simulink model "example_quaternion_KF_EKF"  (R2016a)
settings: Solver=VariableStepAuto  StartTime=0.0  StopTime=25  RelTol=1e-3
values from neighbouring files (symbols this model uses):
  filterMat = filterMat(filterPlot,:)    [init.m]
  KF_C = KF_C([3,4,5,7,8,9,10,11,12,13],:)    [init.m]
  KF_mean = zeros(13,1)    [init.m]
  KF_variance = diag([0.00025, 0.049,0.049,0.05, 0.05, 0.05, 0.05, 0.005, 0.005,0.005])    [init.m]
  measureMat = measureMat(measurePlot,:)    [init.m]
undefined symbols (not defined in the file or in its folder): g, inner_h, k, m
settings Model: Creator=Daniel  LastModifiedBy=mgreiff
settings DataIOCC: LimitDataPoints=on
settings DebuggingCC: AllowSymbolicDim=off
settings ModelReferenceCC: PropagateSignalLabelsOutOfModel=off
settings GRTTargetCC: GeneratePreprocessorConditionals=Use local settings

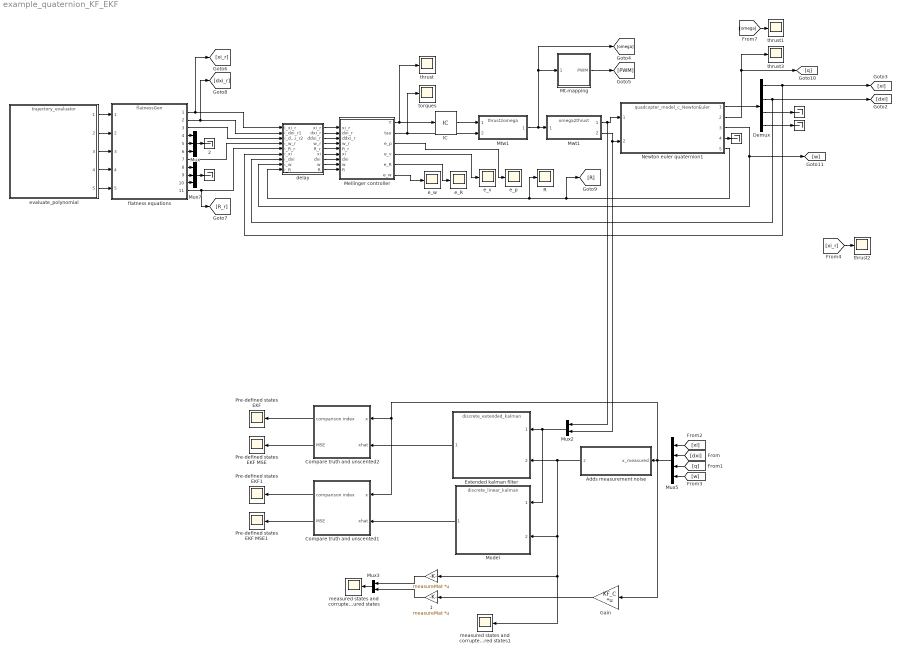
== system example_quaternion_KF_EKF ==
  " " : Gain  Gain=measureMat  Multiplication=Matrix(K*u)
  "  " : Terminator
  "     " : Terminator
  "      " : Terminator
  "       " : Terminator
  " 1" : Gain  Gain=measureMat  Multiplication=Matrix(K*u)
  " 2" : Terminator
  Adds measurement noise : Subsystem
  Compare truth and unscented1 : Subsystem
  Compare truth and unscented2 : Subsystem
  Demux : Demux  Outputs=[3,3,3,3]
  Extended kalman filter : ModelReference  ModelNameDialog=discrete_extended_kalman.slx  SimulationMode=Normal  ModelReferenceVersion=1.22
  Gain : Gain  Gain=KF_C  Multiplication=Matrix(K*u)
  IC : InitialCondition  Value=m*g
  Mellinger controller : MATLAB Function  TreatAsAtomicUnit=on  SystemSampleTime=inner_h
  Model : ModelReference  ModelNameDialog=discrete_linear_kalman.slx  SimulationMode=Normal  ModelReferenceVersion=1.93
  Mt-mapping : Subsystem
  Mtw1 : ModelReference  ModelNameDialog=thrust2omega.mdl  SimulationMode=Normal  ModelReferenceVersion=1.3
  Mux : Mux  Inputs=3
  Mux2 : Mux  Inputs=2
  Mux3 : Mux  Inputs=2
  Mux5 : Mux
  Mux7 : Mux  Inputs=3
  Mwt1 : ModelReference  ModelNameDialog=omega2thrust.mdl  SimulationMode=Normal  ModelReferenceVersion=1.3
  Newton euler quaternion1 : ModelReference  ModelNameDialog=quadcopter_model_c_NewtonEuler.mdl  SimulationMode=Normal  ModelReferenceVersion=1.325
  Pre-defined states EKF : Scope
  Pre-defined states EKF MSE : Scope
  Pre-defined states EKF MSE1 : Scope
  Pre-defined states EKF1 : Scope
  R : Scope
  delay : Subsystem
  e_R : Scope
  e_p : Scope
  e_v : Scope
  e_w : Scope
  evaluate_polynomial : ModelReference  ModelNameDialog=trajectory_evaluator.slx  SimulationMode=Normal  ModelReferenceVersion=1.106
  flatness equations : ModelReference  ModelNameDialog=flatnessGen.slx  SimulationMode=Normal  ModelReferenceVersion=1.117
  measured states and corrupted measured states : Scope
  measured states and corrupted measured states1 : Scope
  thrust{,1..3} (4 alike) : Scope
  torques : Scope
  wires:
  Adds measurement noise/1(z) -> Model/2, measured states and corrupted measured states1/1, " "/1, Extended kalman filter/2
  Gain/1 -> " 1"/1
  Mux2/1 -> Model/1, Extended kalman filter/1
  Mux3/1 -> measured states and corrupted measured states/1
  " "/1 -> Mux3/1
  " 1"/1 -> Mux3/2
  Extended kalman filter/1 -> Compare truth and unscented2/2(xhat)
  Compare truth and unscented2/1(comparison index) -> Pre-defined states EKF/1
  Compare truth and unscented2/2(MSE) -> Pre-defined states EKF MSE/1
  Mux5/1 -> Gain/1, Compare truth and unscented1/1(x), Compare truth and unscented2/1(x), Adds measurement noise/1(x_measured)
  [dxi] -> Mux5/2
  [xi] -> Mux5/1
  [q] -> Mux5/3
  [w] -> Mux5/4
  Compare truth and unscented1/1(comparison index) -> Pre-defined states EKF1/1
  Compare truth and unscented1/2(MSE) -> Pre-defined states EKF MSE1/1
  Model/1 -> Compare truth and unscented1/2(xhat)
  Mt-mapping/1(PWM) -> [PWM]
  Mwt1/1 -> Mux2/1, Newton euler quaternion1/1
  Mwt1/2 -> Mux2/2, Newton euler quaternion1/2
  evaluate_polynomial/1 -> flatness equations/1
  evaluate_polynomial/2 -> flatness equations/2
  evaluate_polynomial/3 -> flatness equations/3
  evaluate_polynomial/4 -> flatness equations/4
  evaluate_polynomial/5 -> flatness equations/5
  Mellinger controller/2(tau) -> torques/1, Mtw1/2
  flatness equations/1 -> delay/1(i_xi_r), [xi_r]
  Newton euler quaternion1/1 -> Demux/1
  Newton euler quaternion1/2 -> [q], thrust3/1
  Demux/2 -> delay/7(i_dxi), [dxi]
  Demux/1 -> [xi], delay/6(i_xi)
  Newton euler quaternion1/4 -> "     "/1
  Mux7/1 -> "  "/1
  Mux/1 -> " 2"/1
  flatness equations/8 -> Mux7/1
  flatness equations/9 -> Mux7/2
  flatness equations/10 -> Mux7/3
  flatness equations/4 -> Mux/1
  flatness equations/5 -> Mux/2
  flatness equations/6 -> Mux/3
  flatness equations/7 -> delay/4(i_w_r)
  flatness equations/3 -> delay/3(i_ddxi_r2)
  flatness equations/11 -> delay/5(i_R_r), [R_r]
  flatness equations/2 -> delay/2(i_dxi_r1), [dxi_r]
  Newton euler quaternion1/5 -> [R], delay/9(i_R), R/1
  Demux/3 -> "      "/1
  Demux/4 -> "       "/1
  Mellinger controller/6(e_w) -> e_w/1
  Mellinger controller/5(e_R) -> e_R/1
  Mellinger controller/4(e_v) -> e_v/1
  Mellinger controller/3(e_p) -> e_p/1
  [omega] -> thrust1/1
  Newton euler quaternion1/3 -> [w], delay/8(i_w)
  delay/1(xi_r) -> Mellinger controller/1(xi_r)
  delay/2(dxi_r) -> Mellinger controller/2(dxi_r)
  delay/3(ddxi_r) -> Mellinger controller/3(ddxi_r)
  delay/4(w_r) -> Mellinger controller/4(w_r)
  delay/5(R_r) -> Mellinger controller/5(R_r)
  delay/6(xi) -> Mellinger controller/6(xi)
  delay/7(dxi) -> Mellinger controller/7(dxi)
  delay/8(w) -> Mellinger controller/8(w)
  delay/9(R) -> Mellinger controller/9(R)
  Mellinger controller/1(T) -> IC/1, thrust/1
  Mtw1/1 -> Mt-mapping/1(omega), [omega], Mwt1/1
  [xi_r] -> thrust2/1
  IC/1 -> Mtw1/1

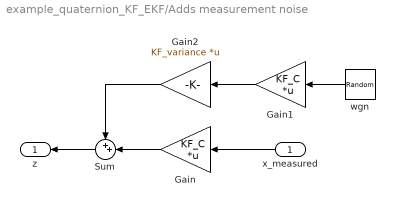
== system example_quaternion_KF_EKF/Adds measurement noise ==
  x_measured : Inport
  Gain : Gain  Gain=KF_C  Multiplication=Matrix(K*u)
  Gain1 : Gain  Gain=KF_C  Multiplication=Matrix(K*u)
  Gain2 : Gain  Gain=KF_variance  Multiplication=Matrix(K*u)
  Sum : Sum  Inputs=++|
  wgn : RandomNumber  Mean=KF_mean
  z : Outport
  wires:
  x_measured/1 -> Gain/1
  Gain1/1 -> Gain2/1
  Sum/1 -> z/1
  Gain/1 -> Sum/2
  Gain2/1 -> Sum/1
  wgn/1 -> Gain1/1

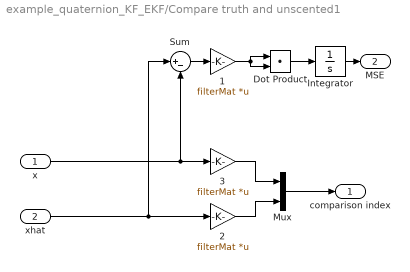
== system example_quaternion_KF_EKF/Compare truth and unscented1 ==
  x : Inport
  xhat : Inport  Port=2
  " 1" : Gain  Gain=filterMat  Multiplication=Matrix(K*u)
  " 2" : Gain  Gain=filterMat  Multiplication=Matrix(K*u)
  " 3" : Gain  Gain=filterMat  Multiplication=Matrix(K*u)
  Dot Product : DotProduct  InputSameDT=on  OutDataTypeStr=Inherit: Inherit via internal rule
  Integrator : Integrator
  Mux : Mux  Inputs=2
  Sum : Sum  Inputs=|+-
  comparison index : Outport
  MSE : Outport  Port=2
  wires:
  xhat/1 -> Sum/1, " 2"/1
  x/1 -> Sum/2, " 3"/1
  " 3"/1 -> Mux/1
  " 2"/1 -> Mux/2
  Mux/1 -> comparison index/1
  " 1"/1 -> Dot Product/2, Dot Product/1
  Dot Product/1 -> Integrator/1
  Sum/1 -> " 1"/1
  Integrator/1 -> MSE/1

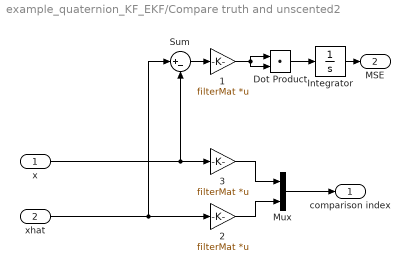
== system example_quaternion_KF_EKF/Compare truth and unscented2 ==
  x : Inport
  xhat : Inport  Port=2
  " 1" : Gain  Gain=filterMat  Multiplication=Matrix(K*u)
  " 2" : Gain  Gain=filterMat  Multiplication=Matrix(K*u)
  " 3" : Gain  Gain=filterMat  Multiplication=Matrix(K*u)
  Dot Product : DotProduct  InputSameDT=on  OutDataTypeStr=Inherit: Inherit via internal rule
  Integrator : Integrator
  Mux : Mux  Inputs=2
  Sum : Sum  Inputs=|+-
  comparison index : Outport
  MSE : Outport  Port=2
  wires:
  xhat/1 -> Sum/1, " 2"/1
  x/1 -> Sum/2, " 3"/1
  " 3"/1 -> Mux/1
  " 2"/1 -> Mux/2
  Mux/1 -> comparison index/1
  " 1"/1 -> Dot Product/2, Dot Product/1
  Dot Product/1 -> Integrator/1
  Sum/1 -> " 1"/1
  Integrator/1 -> MSE/1

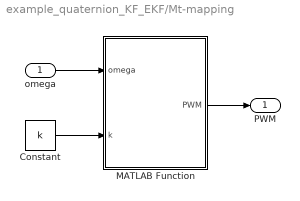
== system example_quaternion_KF_EKF/Mt-mapping ==
  omega : Inport
  Constant : Constant  Value=k
  MATLAB Function : MATLAB Function  TreatAsAtomicUnit=on
  PWM : Outport
  wires:
  MATLAB Function/1(PWM) -> PWM/1
  omega/1 -> MATLAB Function/1(omega)
  Constant/1 -> MATLAB Function/2(k)

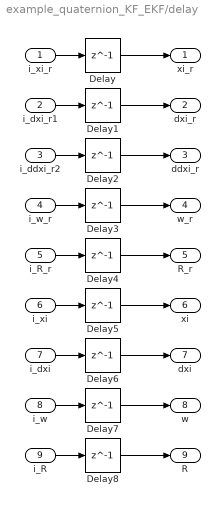
== system example_quaternion_KF_EKF/delay ==
  i_xi_r : Inport
  i_dxi_r1 : Inport  Port=2
  i_ddxi_r2 : Inport  Port=3
  i_w_r : Inport  Port=4
  i_R_r : Inport  Port=5
  i_xi : Inport  Port=6
  i_dxi : Inport  Port=7
  i_w : Inport  Port=8
  i_R : Inport  Port=9
  Delay{,1..8} (9 alike) : Delay  DelayLength=1  InitialCondition=0  SampleTime=inner_h
  xi_r : Outport
  dxi_r : Outport  Port=2
  ddxi_r : Outport  Port=3
  w_r : Outport  Port=4
  R_r : Outport  Port=5
  xi : Outport  Port=6
  dxi : Outport  Port=7
  w : Outport  Port=8
  R : Outport  Port=9
  wires:
  Delay/1 -> xi_r/1
  Delay1/1 -> dxi_r/1
  Delay2/1 -> ddxi_r/1
  Delay4/1 -> R_r/1
  Delay3/1 -> w_r/1
  Delay5/1 -> xi/1
  Delay6/1 -> dxi/1
  Delay8/1 -> R/1
  Delay7/1 -> w/1
  i_xi_r/1 -> Delay/1
  i_ddxi_r2/1 -> Delay2/1
  i_dxi_r1/1 -> Delay1/1
  i_w_r/1 -> Delay3/1
  i_R_r/1 -> Delay4/1
  i_xi/1 -> Delay5/1
  i_dxi/1 -> Delay6/1
  i_w/1 -> Delay7/1
  i_R/1 -> Delay8/1

== matlab function example_quaternion_KF_EKF/Mellinger controller ==
  data: xi_r input; dxi_r input; ddxi_r input; w_r input; R_r input; xi input; T output; tau output; dxi input; w input; R input; e_p output; e_v output; e_R output; e_w output
function [T, tau, e_p, e_v, e_R, e_w] = controller(xi_r, dxi_r, ddxi_r, w_r, R_r, xi, dxi, w, R)
%I = [0.0820; 0.0845; 0.1377];
%A=[0;0;0]
%m = 4.34;

m = 0.027;
g = 9.81;
% Functional tuning for type A
K_p = 0.2 * eye(3);
K_v = 0.025 * eye(3);
K_R = 0.1 * eye(3);
K_w = 0.001 * eye(3);

% Functional tuning for type B
K_p = 0.4 * eye(3);
K_v = 0.1* eye(3);
K_R = 0.4 * eye(3);
K_w = 0.01 * eye(3);

K_p = 0.8 * eye(3);
K_v = 0.12* eye(3);
K_R = 0.5 * eye(3);
K_w = 0.005 * eye(3);

%#codegen
zw = [0; 0; 1];
zb = R(:,3);

e_p = xi_r - xi;
e_v = dxi_r - dxi;
F_des = K_p * e_p + K_v * e_v + m * g * zw + m * ddxi_r;
T = F_des'*zb;

zb_des = F_des./ norm(F_des);
psi = 0;
yc_des = [cos(psi+pi/2); sin(psi+pi/2); 0];
xb_des = cross(yc_des, zb_des)./norm(cross(yc_des, zb_des));
yb_des = cross(zb_des, xb_des);
R_des = [xb_des, yb_des, zb_des];

Ssym = 0.5.* (R_des' * R - R' * R_des);
e_R = -[Ssym(3,2); Ssym(1,3); Ssym(2,1)]; % Vee map
e_w = (w_r - w);

%disp([norm(e_p), norm(e_v), norm(e_R), norm(e_w)])

tau = K_R * e_R + K_w * e_w;

== matlab function example_quaternion_KF_EKF/Mt-mapping/MATLAB Function ==
  data: omega input; PWM output; k input
function PWM = Mt(omega, k)
%#codegen
rotor_thrusts = k.*omega.^2;
beta1 = 0.0877;
beta2 = 0.0660;
PWM =  -beta1/(2*beta2) + sqrt((beta1/(2*beta2))^2 + rotor_thrusts/beta2);
